simulink model "attsync"  (R2013b)
settings: Solver=ode45  StartTime=0.0  StopTime=100  RelTol=1e-3
settings Model: Creator=daqing_yi  LastModifiedBy=Walter
settings DataIOCC: SignalLoggingSaveFormat=ModelDataLogs
settings DebuggingCC: MultiTaskDSMMsg=warning  MultiTaskCondExecSysMsg=none  StateNameClashWarn=warning
settings RTWCC: IncludeERTFirstTime=on

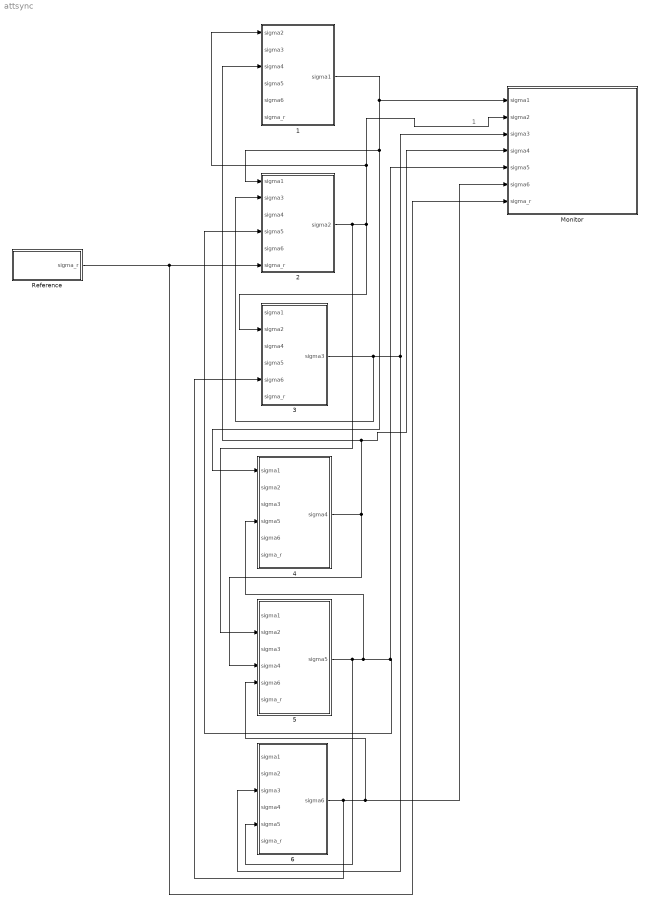
== system attsync ==
  note: 1
  1 : Subsystem
  2 : Subsystem
  3 : Subsystem
  4 : Subsystem
  5 : Subsystem
  6 : Subsystem
  Monitor : Subsystem
  Reference : Subsystem
  wires:
  3/1(sigma3) -> 2/2(sigma3), 6/3(sigma3), Monitor/3(sigma3)
  4/1(sigma4) -> Monitor/4(sigma4), 1/3(sigma4), 5/4(sigma4)
  5/1(sigma5) -> 6/5(sigma5), 4/4(sigma5), Monitor/5(sigma5), 2/4(sigma5)
  6/1(sigma6) -> 3/5(sigma6), 5/5(sigma6), Monitor/6(sigma6)
  Reference/1(sigma_r) -> Monitor/7(sigma_r), 2/6(sigma_r)
  2/1(sigma2) -> 5/2(sigma2), Monitor/2(sigma2), 1/1(sigma2), 3/2(sigma2)
  1/1(sigma1) -> 4/1(sigma1), 2/1(sigma1), Monitor/1(sigma1)

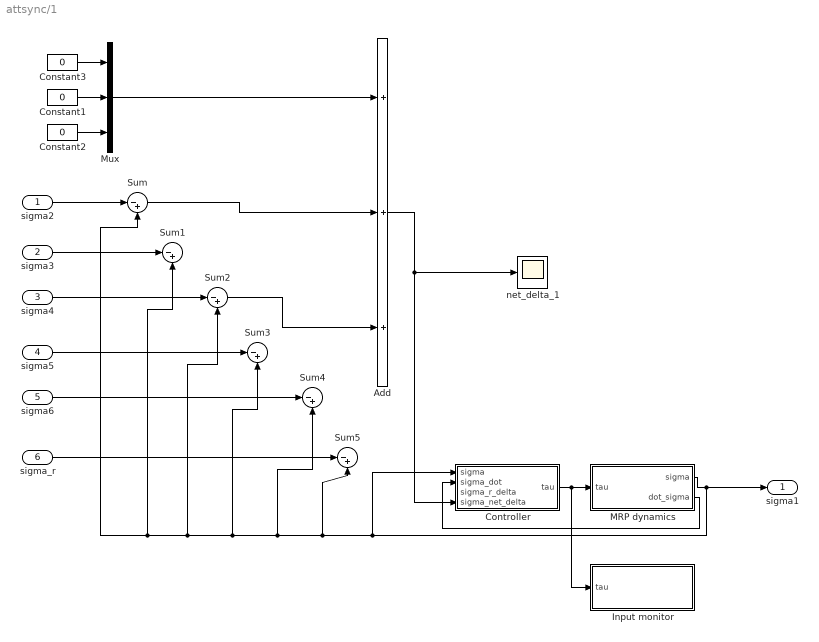
== system attsync/1 ==
  sigma2 : Inport  PortDimensions=3
  sigma3 : Inport  Port=2  PortDimensions=3
  sigma4 : Inport  Port=3  PortDimensions=3
  sigma5 : Inport  Port=4  PortDimensions=3
  sigma6 : Inport  Port=5  PortDimensions=3
  sigma_r : Inport  Port=6  PortDimensions=3
  Add : Sum  Inputs=+++
  Constant1 : Constant  Value=0
  Constant2 : Constant  Value=0
  Constant3 : Constant  Value=0
  Controller : Subsystem
  Input monitor : Subsystem
  MRP dynamics : Subsystem
  Mux : Mux  Inputs=3
  Sum{,1..5} (6 alike) : Sum  Inputs=|-+
  net_delta_1 : Scope
      settings: SaveName=ScopeData7
  sigma1 : Outport
  wires:
  Controller/1(tau) -> Input monitor/1(tau), MRP dynamics/1(tau)
  MRP dynamics/1(sigma) -> sigma1/1, Sum5/2, Sum/2, Sum1/2, Sum2/2, Sum3/2, Sum4/2, Controller/1(sigma)
  sigma6/1 -> Sum4/1
  sigma5/1 -> Sum3/1
  sigma4/1 -> Sum2/1
  sigma3/1 -> Sum1/1
  sigma2/1 -> Sum/1
  Add/1 -> net_delta_1/1, Controller/4("sigma_net_delta ")
  Mux/1 -> Add/1
  Constant3/1 -> Mux/1
  Constant1/1 -> Mux/2
  Constant2/1 -> Mux/3
  Sum2/1 -> Add/3
  Sum/1 -> Add/2
  sigma_r/1 -> Sum5/1
  MRP dynamics/2(dot_sigma) -> Controller/2(sigma_dot)

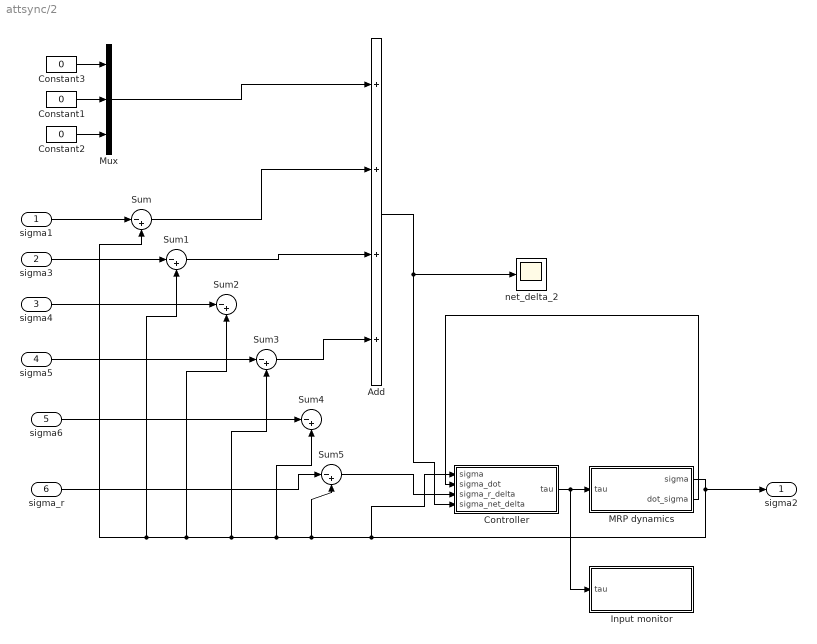
== system attsync/2 ==
  sigma1 : Inport  PortDimensions=3
  sigma3 : Inport  Port=2  PortDimensions=3
  sigma4 : Inport  Port=3  PortDimensions=3
  sigma5 : Inport  Port=4  PortDimensions=3
  sigma6 : Inport  Port=5  PortDimensions=3
  sigma_r : Inport  Port=6  PortDimensions=3
  Add : Sum  Inputs=++++
  Constant1 : Constant  Value=0
  Constant2 : Constant  Value=0
  Constant3 : Constant  Value=0
  Controller : Subsystem
  Input monitor : Subsystem
  MRP dynamics : Subsystem
  Mux : Mux  Inputs=3
  Sum{,1..5} (6 alike) : Sum  Inputs=|-+
  net_delta_2 : Scope
      settings: SaveName=ScopeData7
  sigma2 : Outport
  wires:
  Controller/1(tau) -> MRP dynamics/1(tau), Input monitor/1(tau)
  sigma6/1 -> Sum4/1
  sigma5/1 -> Sum3/1
  sigma4/1 -> Sum2/1
  sigma3/1 -> Sum1/1
  sigma1/1 -> Sum/1
  Add/1 -> Controller/4("sigma_net_delta "), net_delta_2/1
  Mux/1 -> Add/1
  Constant3/1 -> Mux/1
  Constant1/1 -> Mux/2
  Constant2/1 -> Mux/3
  Sum/1 -> Add/2
  Sum3/1 -> Add/4
  Sum1/1 -> Add/3
  sigma_r/1 -> Sum5/1
  Sum5/1 -> Controller/3(sigma_r_delta)
  MRP dynamics/2(dot_sigma) -> Controller/2(sigma_dot)
  MRP dynamics/1(sigma) -> sigma2/1, Controller/1(sigma), Sum5/2, Sum/2, Sum1/2, Sum2/2, Sum3/2, Sum4/2

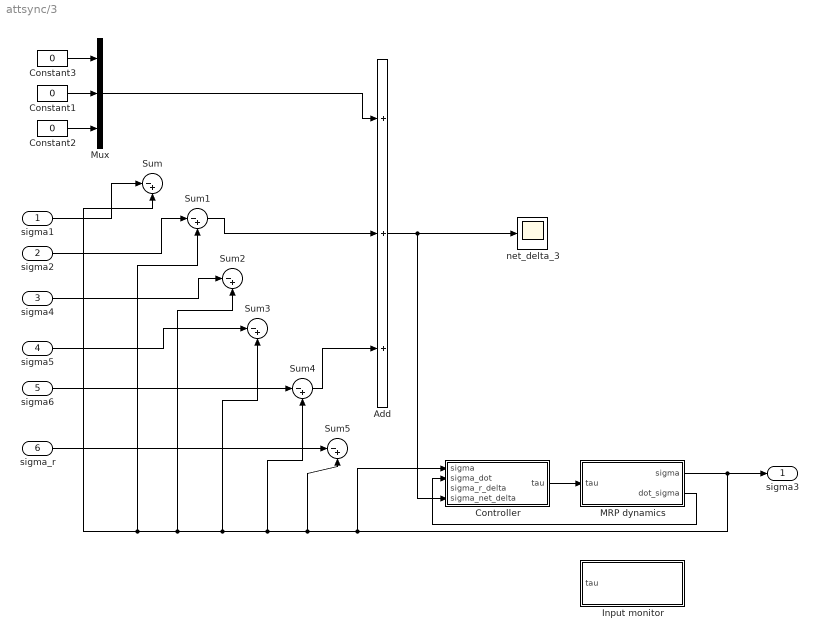
== system attsync/3 ==
  sigma1 : Inport  PortDimensions=3
  sigma2 : Inport  Port=2  PortDimensions=3
  sigma4 : Inport  Port=3  PortDimensions=3
  sigma5 : Inport  Port=4  PortDimensions=3
  sigma6 : Inport  Port=5  PortDimensions=3
  sigma_r : Inport  Port=6  PortDimensions=3
  Add : Sum  Inputs=+++
  Constant1 : Constant  Value=0
  Constant2 : Constant  Value=0
  Constant3 : Constant  Value=0
  Controller : Subsystem
  Input monitor : Subsystem
  MRP dynamics : Subsystem
  Mux : Mux  Inputs=3
  Sum{,1..5} (6 alike) : Sum  Inputs=|-+
  net_delta_3 : Scope
      settings: SaveName=ScopeData7
  sigma3 : Outport
  wires:
  Controller/1(tau) -> MRP dynamics/1(tau)
  MRP dynamics/1(sigma) -> Controller/1(sigma), Sum5/2, Sum/2, Sum1/2, Sum2/2, Sum3/2, Sum4/2, sigma3/1
  sigma6/1 -> Sum4/1
  sigma5/1 -> Sum3/1
  sigma4/1 -> Sum2/1
  sigma2/1 -> Sum1/1
  sigma1/1 -> Sum/1
  Add/1 -> Controller/4("sigma_net_delta "), net_delta_3/1
  Mux/1 -> Add/1
  Constant3/1 -> Mux/1
  Constant1/1 -> Mux/2
  Constant2/1 -> Mux/3
  Sum1/1 -> Add/2
  Sum4/1 -> Add/3
  sigma_r/1 -> Sum5/1
  MRP dynamics/2(dot_sigma) -> Controller/2(sigma_dot)

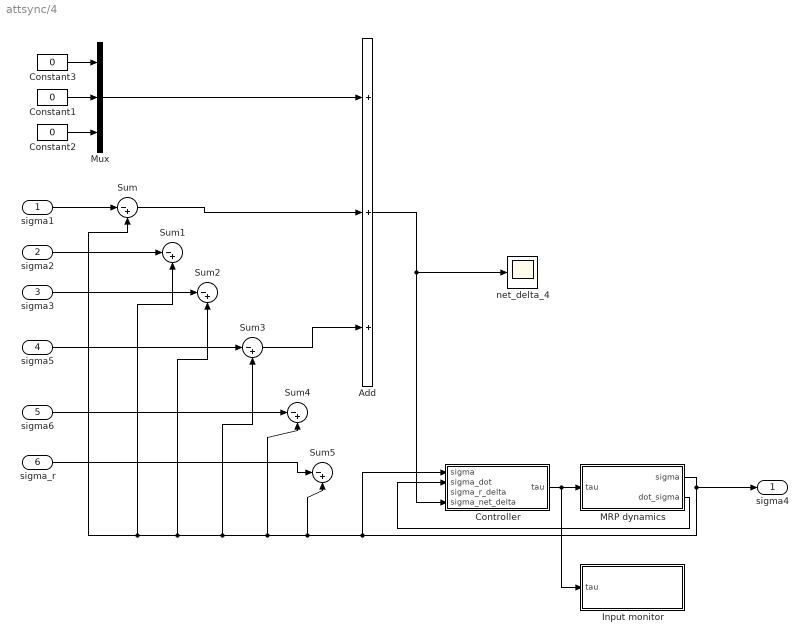
== system attsync/4 ==
  sigma1 : Inport  PortDimensions=3
  sigma2 : Inport  Port=2  PortDimensions=3
  sigma3 : Inport  Port=3  PortDimensions=3
  sigma5 : Inport  Port=4  PortDimensions=3
  sigma6 : Inport  Port=5  PortDimensions=3
  sigma_r : Inport  Port=6  PortDimensions=3
  Add : Sum  Inputs=+++
  Constant1 : Constant  Value=0
  Constant2 : Constant  Value=0
  Constant3 : Constant  Value=0
  Controller : Subsystem
  Input monitor : Subsystem
  MRP dynamics : Subsystem
  Mux : Mux  Inputs=3
  Sum{,1..5} (6 alike) : Sum  Inputs=|-+
  net_delta_4 : Scope
      settings: SaveName=ScopeData7
  sigma4 : Outport
  wires:
  Controller/1(tau) -> MRP dynamics/1(tau), Input monitor/1(tau)
  MRP dynamics/1(sigma) -> sigma4/1, Controller/1(sigma), Sum5/2, Sum/2, Sum1/2, Sum2/2, Sum3/2, Sum4/2
  sigma6/1 -> Sum4/1
  sigma5/1 -> Sum3/1
  sigma3/1 -> Sum2/1
  sigma2/1 -> Sum1/1
  sigma1/1 -> Sum/1
  Add/1 -> Controller/4("sigma_net_delta "), net_delta_4/1
  Mux/1 -> Add/1
  Constant3/1 -> Mux/1
  Constant1/1 -> Mux/2
  Constant2/1 -> Mux/3
  Sum/1 -> Add/2
  Sum3/1 -> Add/3
  sigma_r/1 -> Sum5/1
  MRP dynamics/2(dot_sigma) -> Controller/2(sigma_dot)

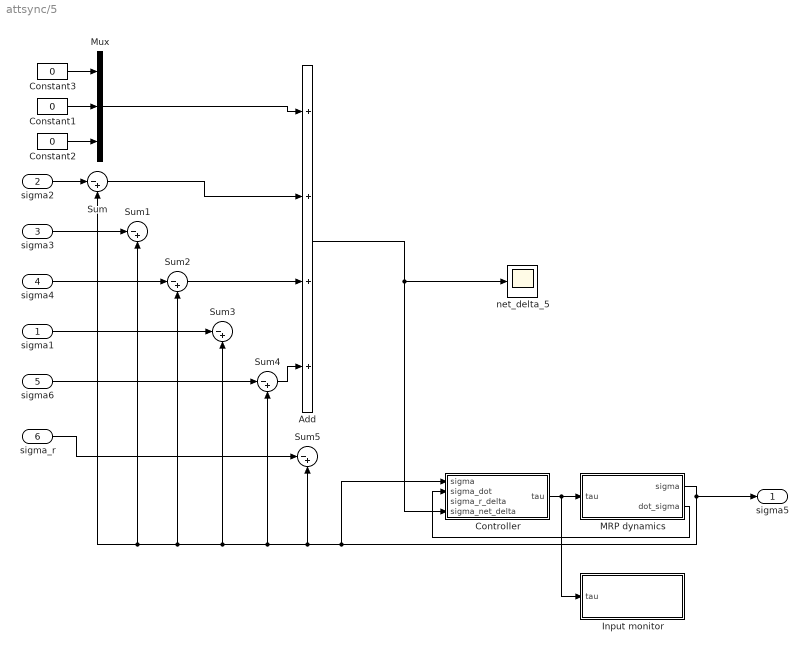
== system attsync/5 ==
  sigma1 : Inport  PortDimensions=3
  sigma2 : Inport  Port=2  PortDimensions=3
  sigma3 : Inport  Port=3  PortDimensions=3
  sigma4 : Inport  Port=4  PortDimensions=3
  sigma6 : Inport  Port=5  PortDimensions=3
  sigma_r : Inport  Port=6  PortDimensions=3
  Add : Sum  Inputs=++++
  Constant1 : Constant  Value=0
  Constant2 : Constant  Value=0
  Constant3 : Constant  Value=0
  Controller : Subsystem
  Input monitor : Subsystem
  MRP dynamics : Subsystem
  Mux : Mux  Inputs=3
  Sum{,1..5} (6 alike) : Sum  Inputs=|-+
  net_delta_5 : Scope
      settings: SaveName=ScopeData7
  sigma5 : Outport
  wires:
  Controller/1(tau) -> MRP dynamics/1(tau), Input monitor/1(tau)
  sigma6/1 -> Sum4/1
  sigma1/1 -> Sum3/1
  sigma4/1 -> Sum2/1
  sigma3/1 -> Sum1/1
  sigma2/1 -> Sum/1
  Add/1 -> Controller/4("sigma_net_delta "), net_delta_5/1
  Mux/1 -> Add/1
  Constant3/1 -> Mux/1
  Constant1/1 -> Mux/2
  Constant2/1 -> Mux/3
  Sum/1 -> Add/2
  Sum2/1 -> Add/3
  Sum4/1 -> Add/4
  sigma_r/1 -> Sum5/1
  MRP dynamics/1(sigma) -> sigma5/1, Controller/1(sigma), Sum5/2, Sum/2, Sum1/2, Sum2/2, Sum3/2, Sum4/2
  MRP dynamics/2(dot_sigma) -> Controller/2(sigma_dot)

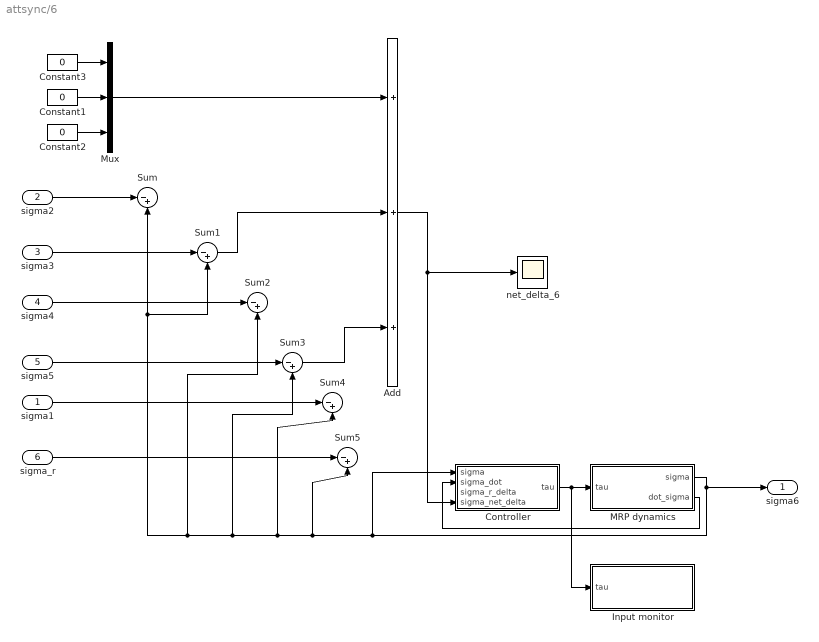
== system attsync/6 ==
  sigma1 : Inport  PortDimensions=3
  sigma2 : Inport  Port=2  PortDimensions=3
  sigma3 : Inport  Port=3  PortDimensions=3
  sigma4 : Inport  Port=4  PortDimensions=3
  sigma5 : Inport  Port=5  PortDimensions=3
  sigma_r : Inport  Port=6  PortDimensions=3
  Add : Sum  Inputs=+++
  Constant1 : Constant  Value=0
  Constant2 : Constant  Value=0
  Constant3 : Constant  Value=0
  Controller : Subsystem
  Input monitor : Subsystem
  MRP dynamics : Subsystem
  Mux : Mux  Inputs=3
  Sum{,1..5} (6 alike) : Sum  Inputs=|-+
  net_delta_6 : Scope
      settings: SaveName=ScopeData7
  sigma6 : Outport
  wires:
  Controller/1(tau) -> MRP dynamics/1(tau), Input monitor/1(tau)
  MRP dynamics/1(sigma) -> sigma6/1, Controller/1(sigma), Sum5/2, Sum/2, Sum1/2, Sum2/2, Sum3/2, Sum4/2
  sigma1/1 -> Sum4/1
  sigma5/1 -> Sum3/1
  sigma4/1 -> Sum2/1
  sigma3/1 -> Sum1/1
  sigma2/1 -> Sum/1
  Add/1 -> Controller/4("sigma_net_delta "), net_delta_6/1
  Mux/1 -> Add/1
  Constant3/1 -> Mux/1
  Constant1/1 -> Mux/2
  Constant2/1 -> Mux/3
  Sum1/1 -> Add/2
  Sum3/1 -> Add/3
  sigma_r/1 -> Sum5/1
  MRP dynamics/2(dot_sigma) -> Controller/2(sigma_dot)

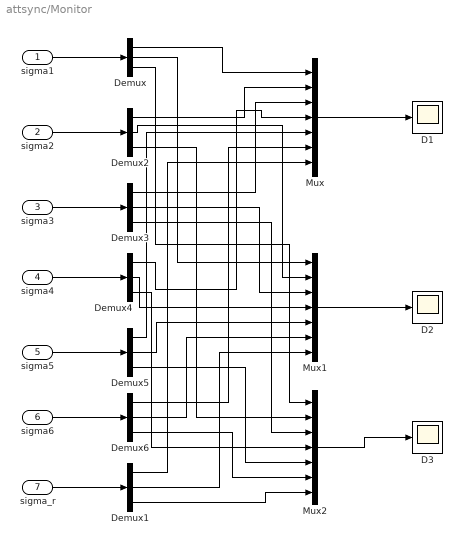
== system attsync/Monitor ==
  sigma1 : Inport
  sigma2 : Inport  Port=2
  sigma3 : Inport  Port=3
  sigma4 : Inport  Port=4
  sigma5 : Inport  Port=5
  sigma6 : Inport  Port=6
  sigma_r : Inport  Port=7
  D1 : Scope
      settings: ShowLegends=on  YMin=1.75  YMax=2.025  SaveName=D1
  "D2 " : Scope
      settings: SaveName=D2
  D3 : Scope
      settings: SaveName=D3
  Demux{,1..6} (7 alike) : Demux  Outputs=3
  Mux : Mux  Inputs=7
  Mux1 : Mux  Inputs=7
  Mux2 : Mux  Inputs=7
  wires:
  sigma1/1 -> Demux/1
  Demux/1 -> Mux/1
  Demux1/1 -> Mux/7
  Demux/2 -> Mux1/1
  Demux1/2 -> Mux1/7
  Demux/3 -> Mux2/1
  Demux1/3 -> Mux2/7
  sigma_r/1 -> Demux1/1
  sigma6/1 -> Demux6/1
  sigma5/1 -> Demux5/1
  sigma4/1 -> Demux4/1
  sigma3/1 -> Demux3/1
  sigma2/1 -> Demux2/1
  Demux2/1 -> Mux/2
  Demux3/1 -> Mux/3
  Demux4/1 -> Mux/4
  Demux2/2 -> Mux1/2
  Demux5/1 -> Mux/5
  Demux6/1 -> Mux/6
  Demux4/2 -> Mux1/4
  Demux3/2 -> Mux1/3
  Demux5/2 -> Mux1/5
  Demux6/2 -> Mux1/6
  Demux2/3 -> Mux2/2
  Demux3/3 -> Mux2/3
  Demux4/3 -> Mux2/4
  Demux5/3 -> Mux2/5
  Demux6/3 -> Mux2/6
  Mux2/1 -> D3/1
  Mux1/1 -> "D2 "/1
  Mux/1 -> D1/1

== system attsync/Reference ==
  Constant1 : Constant  Value=1.5
  Constant2 : Constant
  Constant3 : Constant  Value=2
  Mux : Mux  Inputs=3
  sigma_r : Outport
  wires:
  Mux/1 -> sigma_r/1
  Constant3/1 -> Mux/1
  Constant1/1 -> Mux/2
  Constant2/1 -> Mux/3

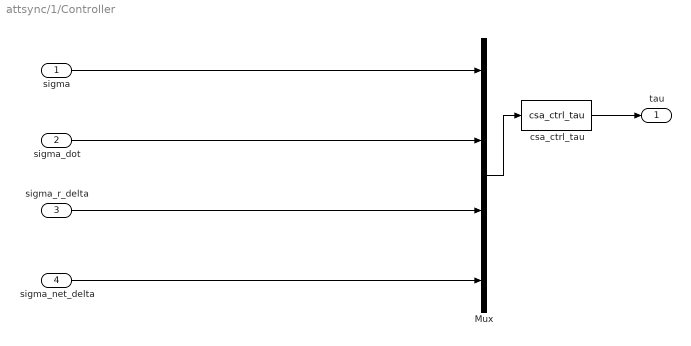
== system attsync/1/Controller ==
  sigma : Inport  PortDimensions=3
  sigma_dot : Inport  Port=2
  sigma_r_delta : Inport  Port=3  PortDimensions=3
  "sigma_net_delta " : Inport  Port=4  PortDimensions=3
  Mux : Mux
  csa_ctrl_tau : MATLABFcn  MATLABFcn=csa_ctrl_tau
  tau : Outport
  wires:
  sigma/1 -> Mux/1
  Mux/1 -> csa_ctrl_tau/1
  csa_ctrl_tau/1 -> tau/1
  sigma_r_delta/1 -> Mux/3
  "sigma_net_delta "/1 -> Mux/4
  sigma_dot/1 -> Mux/2

== system attsync/1/Input monitor ==
  tau : Inport
  Demux : Demux  Outputs=3
  tau1 : Scope
      settings: SaveName=ScopeData3
  tau2 : Scope
      settings: SaveName=ScopeData4
  tau3 : Scope
      settings: SaveName=ScopeData5
  wires:
  Demux/1 -> tau1/1
  Demux/2 -> tau2/1
  Demux/3 -> tau3/1
  tau/1 -> Demux/1

== system attsync/1/MRP dynamics ==
  tau : Inport
  Demux : Demux  Outputs=2
  S-Function : S-Function  FunctionName=mrp_dynamics1  EnableBusSupport=off
  sigma : Outport  PortDimensions=3
  dot_sigma : Outport  Port=2  PortDimensions=3
  wires:
  tau/1 -> S-Function/1
  S-Function/1 -> Demux/1
  Demux/1 -> sigma/1
  Demux/2 -> dot_sigma/1

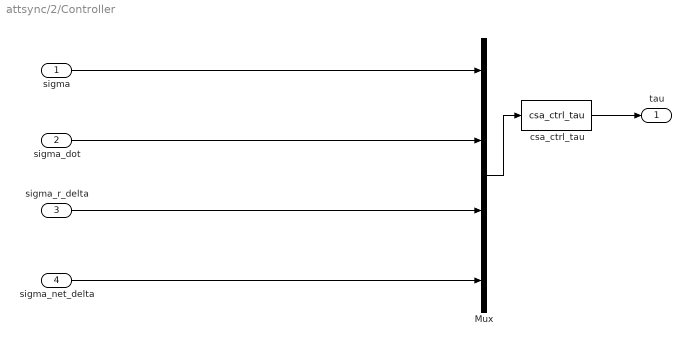
== system attsync/2/Controller ==
  sigma : Inport  PortDimensions=3
  sigma_dot : Inport  Port=2
  sigma_r_delta : Inport  Port=3  PortDimensions=3
  "sigma_net_delta " : Inport  Port=4  PortDimensions=3
  Mux : Mux
  csa_ctrl_tau : MATLABFcn  MATLABFcn=csa_ctrl_tau
  tau : Outport
  wires:
  sigma/1 -> Mux/1
  Mux/1 -> csa_ctrl_tau/1
  csa_ctrl_tau/1 -> tau/1
  sigma_r_delta/1 -> Mux/3
  "sigma_net_delta "/1 -> Mux/4
  sigma_dot/1 -> Mux/2

== system attsync/2/Input monitor ==
  tau : Inport
  Demux : Demux  Outputs=3
  tau1 : Scope
      settings: SaveName=ScopeData3
  tau2 : Scope
      settings: SaveName=ScopeData4
  tau3 : Scope
      settings: SaveName=ScopeData5
  wires:
  Demux/1 -> tau1/1
  Demux/2 -> tau2/1
  Demux/3 -> tau3/1
  tau/1 -> Demux/1

== system attsync/2/MRP dynamics ==
  tau : Inport
  Demux : Demux  Outputs=2
  S-Function : S-Function  FunctionName=mrp_dynamics2  EnableBusSupport=off
  sigma : Outport  PortDimensions=3
  dot_sigma : Outport  Port=2  PortDimensions=3
  wires:
  tau/1 -> S-Function/1
  S-Function/1 -> Demux/1
  Demux/1 -> sigma/1
  Demux/2 -> dot_sigma/1

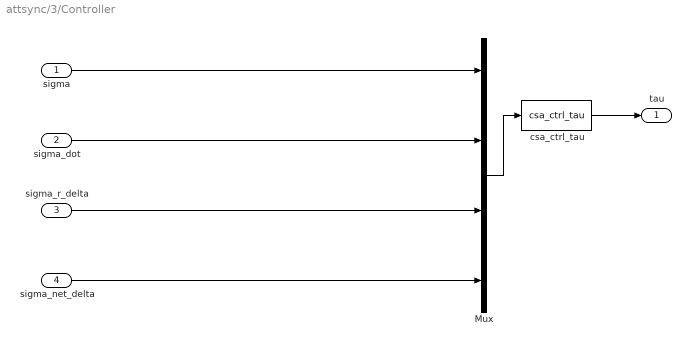
== system attsync/3/Controller ==
  sigma : Inport  PortDimensions=3
  sigma_dot : Inport  Port=2
  sigma_r_delta : Inport  Port=3  PortDimensions=3
  "sigma_net_delta " : Inport  Port=4  PortDimensions=3
  Mux : Mux
  csa_ctrl_tau : MATLABFcn  MATLABFcn=csa_ctrl_tau
  tau : Outport
  wires:
  sigma/1 -> Mux/1
  Mux/1 -> csa_ctrl_tau/1
  csa_ctrl_tau/1 -> tau/1
  sigma_r_delta/1 -> Mux/3
  "sigma_net_delta "/1 -> Mux/4
  sigma_dot/1 -> Mux/2

== system attsync/3/Input monitor ==
  tau : Inport
  Demux : Demux  Outputs=3
  tau1 : Scope
      settings: SaveName=ScopeData3
  tau2 : Scope
      settings: SaveName=ScopeData4
  tau3 : Scope
      settings: SaveName=ScopeData5
  wires:
  Demux/1 -> tau1/1
  Demux/2 -> tau2/1
  Demux/3 -> tau3/1
  tau/1 -> Demux/1

== system attsync/3/MRP dynamics ==
  tau : Inport
  Demux : Demux  Outputs=2
  S-Function : S-Function  FunctionName=mrp_dynamics3  EnableBusSupport=off
  sigma : Outport  PortDimensions=3
  dot_sigma : Outport  Port=2  PortDimensions=3
  wires:
  tau/1 -> S-Function/1
  S-Function/1 -> Demux/1
  Demux/1 -> sigma/1
  Demux/2 -> dot_sigma/1

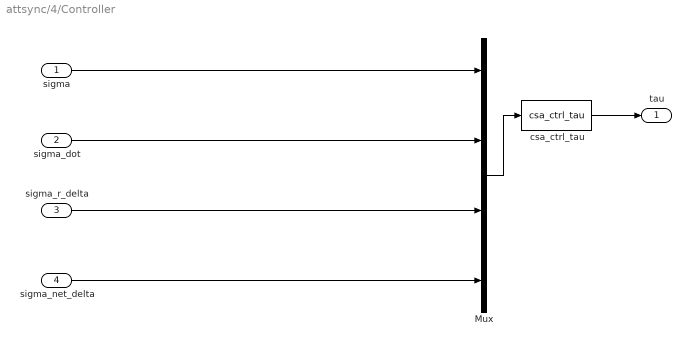
== system attsync/4/Controller ==
  sigma : Inport  PortDimensions=3
  sigma_dot : Inport  Port=2
  sigma_r_delta : Inport  Port=3  PortDimensions=3
  "sigma_net_delta " : Inport  Port=4  PortDimensions=3
  Mux : Mux
  csa_ctrl_tau : MATLABFcn  MATLABFcn=csa_ctrl_tau
  tau : Outport
  wires:
  sigma/1 -> Mux/1
  Mux/1 -> csa_ctrl_tau/1
  csa_ctrl_tau/1 -> tau/1
  sigma_r_delta/1 -> Mux/3
  "sigma_net_delta "/1 -> Mux/4
  sigma_dot/1 -> Mux/2

== system attsync/4/Input monitor ==
  tau : Inport
  Demux : Demux  Outputs=3
  tau1 : Scope
      settings: SaveName=ScopeData3
  tau2 : Scope
      settings: SaveName=ScopeData4
  tau3 : Scope
      settings: SaveName=ScopeData5
  wires:
  Demux/1 -> tau1/1
  Demux/2 -> tau2/1
  Demux/3 -> tau3/1
  tau/1 -> Demux/1

== system attsync/4/MRP dynamics ==
  tau : Inport
  Demux : Demux  Outputs=2
  S-Function : S-Function  FunctionName=mrp_dynamics4  EnableBusSupport=off
  sigma : Outport  PortDimensions=3
  dot_sigma : Outport  Port=2  PortDimensions=3
  wires:
  tau/1 -> S-Function/1
  S-Function/1 -> Demux/1
  Demux/1 -> sigma/1
  Demux/2 -> dot_sigma/1

== system attsync/5/Controller ==
  sigma : Inport
  sigma_dot : Inport  Port=2
  sigma_r_delta : Inport  Port=3  PortDimensions=3
  "sigma_net_delta " : Inport  Port=4  PortDimensions=3
  Mux : Mux
  csa_ctrl_tau : MATLABFcn  MATLABFcn=csa_ctrl_tau
  tau : Outport
  wires:
  sigma/1 -> Mux/1
  Mux/1 -> csa_ctrl_tau/1
  csa_ctrl_tau/1 -> tau/1
  sigma_r_delta/1 -> Mux/3
  "sigma_net_delta "/1 -> Mux/4
  sigma_dot/1 -> Mux/2

== system attsync/5/Input monitor ==
  tau : Inport
  Demux : Demux  Outputs=3
  tau1 : Scope
      settings: SaveName=ScopeData3
  tau2 : Scope
      settings: SaveName=ScopeData4
  tau3 : Scope
      settings: SaveName=ScopeData5
  wires:
  Demux/1 -> tau1/1
  Demux/2 -> tau2/1
  Demux/3 -> tau3/1
  tau/1 -> Demux/1

== system attsync/5/MRP dynamics ==
  tau : Inport
  Demux : Demux  Outputs=2
  S-Function : S-Function  FunctionName=mrp_dynamics5  EnableBusSupport=off
  sigma : Outport  PortDimensions=3
  dot_sigma : Outport  Port=2  PortDimensions=3
  wires:
  tau/1 -> S-Function/1
  S-Function/1 -> Demux/1
  Demux/1 -> sigma/1
  Demux/2 -> dot_sigma/1

== system attsync/6/Controller ==
  sigma : Inport
  sigma_dot : Inport  Port=2
  sigma_r_delta : Inport  Port=3  PortDimensions=3
  "sigma_net_delta " : Inport  Port=4  PortDimensions=3
  Mux : Mux
  csa_ctrl_tau : MATLABFcn  MATLABFcn=csa_ctrl_tau
  tau : Outport
  wires:
  sigma/1 -> Mux/1
  Mux/1 -> csa_ctrl_tau/1
  csa_ctrl_tau/1 -> tau/1
  sigma_r_delta/1 -> Mux/3
  "sigma_net_delta "/1 -> Mux/4
  sigma_dot/1 -> Mux/2

== system attsync/6/Input monitor ==
  tau : Inport
  Demux : Demux  Outputs=3
  tau1 : Scope
      settings: SaveName=ScopeData3
  tau2 : Scope
      settings: SaveName=ScopeData4
  tau3 : Scope
      settings: SaveName=ScopeData5
  wires:
  Demux/1 -> tau1/1
  Demux/2 -> tau2/1
  Demux/3 -> tau3/1
  tau/1 -> Demux/1

== system attsync/6/MRP dynamics ==
  tau : Inport
  Demux : Demux  Outputs=2
  S-Function : S-Function  FunctionName=mrp_dynamics6  EnableBusSupport=off
  sigma : Outport  PortDimensions=3
  dot_sigma : Outport  Port=2  PortDimensions=3
  wires:
  tau/1 -> S-Function/1
  S-Function/1 -> Demux/1
  Demux/1 -> sigma/1
  Demux/2 -> dot_sigma/1
